simulink model "TST_CrCtl_StTrans"  (R2016b)
settings: Solver=FixedStepDiscrete  StartTime=0.0  StopTime=simTime  FixedStep=sampleTime  RelTol=1e-3
values from neighbouring files (symbols this model uses):
  testCase = 1    [initTST_CrCtl_StTrans_001.m]    (also in initTST_CrCtl_StTrans_002.m = 2; initTST_CrCtl_StTrans_003.m = 3; initTST_CrCtl_StTrans_004.m = 4; initTST_CrCtl_StTrans_005.m = 5)
libraries: simulink x46, UnitTest_Lib x5
(part 1 of 2)
settings Model: Creator=shiliwei  LastModifiedBy=shiliwei
settings DebuggingCC: SignalRangeChecking=error

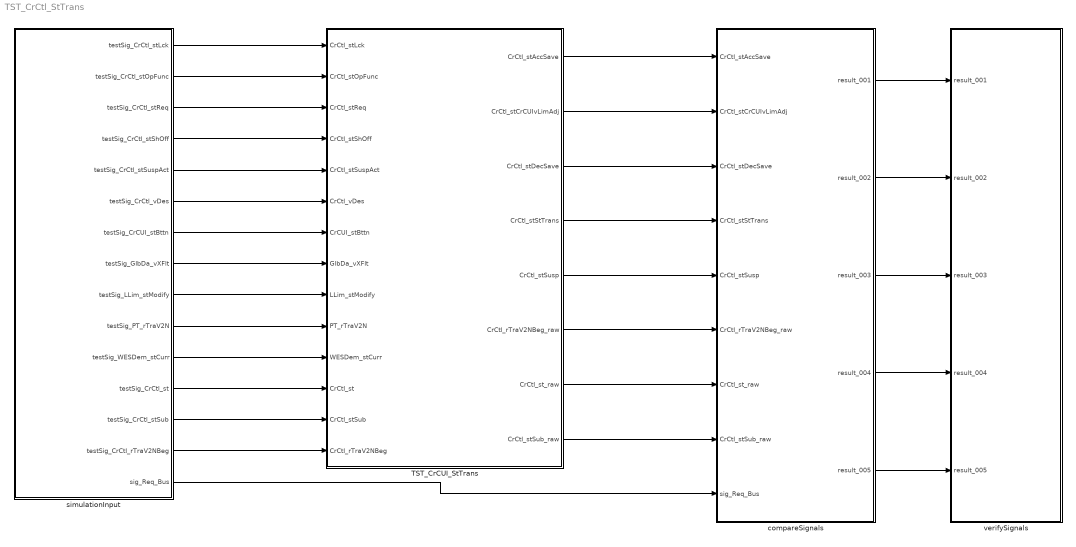
== system TST_CrCtl_StTrans ==
  TST_CrCUI_StTrans : Subsystem
  compareSignals : Subsystem
  simulationInput : Subsystem
  verifySignals : Subsystem
  wires:
  simulationInput/1(testSig_CrCtl_stLck) -> TST_CrCUI_StTrans/1(CrCtl_stLck)
  simulationInput/2(testSig_CrCtl_stOpFunc) -> TST_CrCUI_StTrans/2(CrCtl_stOpFunc)
  simulationInput/3(testSig_CrCtl_stReq) -> TST_CrCUI_StTrans/3(CrCtl_stReq)
  simulationInput/4(testSig_CrCtl_stShOff) -> TST_CrCUI_StTrans/4(CrCtl_stShOff)
  simulationInput/5(testSig_CrCtl_stSuspAct) -> TST_CrCUI_StTrans/5(CrCtl_stSuspAct)
  simulationInput/6(testSig_CrCtl_vDes) -> TST_CrCUI_StTrans/6(CrCtl_vDes)
  simulationInput/7(testSig_CrCUI_stBttn) -> TST_CrCUI_StTrans/7(CrCUI_stBttn)
  simulationInput/8(testSig_GlbDa_vXFlt) -> TST_CrCUI_StTrans/8(GlbDa_vXFlt)
  simulationInput/9(testSig_LLim_stModify) -> TST_CrCUI_StTrans/9(LLim_stModify)
  simulationInput/10(testSig_PT_rTraV2N) -> TST_CrCUI_StTrans/10(PT_rTraV2N)
  simulationInput/11(testSig_WESDem_stCurr) -> TST_CrCUI_StTrans/11(WESDem_stCurr)
  simulationInput/12(testSig_CrCtl_st) -> TST_CrCUI_StTrans/12(CrCtl_st)
  simulationInput/13(testSig_CrCtl_stSub) -> TST_CrCUI_StTrans/13(CrCtl_stSub)
  simulationInput/14(testSig_CrCtl_rTraV2NBeg) -> TST_CrCUI_StTrans/14(CrCtl_rTraV2NBeg)
  TST_CrCUI_StTrans/1(CrCtl_stAccSave) -> compareSignals/1(CrCtl_stAccSave)
  TST_CrCUI_StTrans/2(CrCtl_stCrCUIvLimAdj) -> compareSignals/2(CrCtl_stCrCUIvLimAdj)
  TST_CrCUI_StTrans/3(CrCtl_stDecSave) -> compareSignals/3(CrCtl_stDecSave)
  TST_CrCUI_StTrans/4(CrCtl_stStTrans) -> compareSignals/4(CrCtl_stStTrans)
  TST_CrCUI_StTrans/5(CrCtl_stSusp) -> compareSignals/5(CrCtl_stSusp)
  TST_CrCUI_StTrans/6(CrCtl_rTraV2NBeg_raw) -> compareSignals/6(CrCtl_rTraV2NBeg_raw)
  TST_CrCUI_StTrans/7(CrCtl_st_raw) -> compareSignals/7(CrCtl_st_raw)
  TST_CrCUI_StTrans/8(CrCtl_stSub_raw) -> compareSignals/8(CrCtl_stSub_raw)
  simulationInput/15(sig_Req_Bus) -> compareSignals/9(sig_Req_Bus)
  compareSignals/1(result_001) -> verifySignals/1(result_001)
  compareSignals/2(result_002) -> verifySignals/2(result_002)
  compareSignals/3(result_003) -> verifySignals/3(result_003)
  compareSignals/4(result_004) -> verifySignals/4(result_004)
  compareSignals/5(result_005) -> verifySignals/5(result_005)

== system TST_CrCtl_StTrans/TST_CrCUI_StTrans ==
  CrCtl_stLck : Inport
  CrCtl_stOpFunc : Inport  Port=2
  CrCtl_stReq : Inport  Port=3
  CrCtl_stShOff : Inport  Port=4
  CrCtl_stSuspAct : Inport  Port=5
  CrCtl_vDes : Inport  Port=6
  CrCUI_stBttn : Inport  Port=7
  GlbDa_vXFlt : Inport  Port=8
  LLim_stModify : Inport  Port=9
  PT_rTraV2N : Inport  Port=10
  WESDem_stCurr : Inport  Port=11
  CrCtl_st : Inport  Port=12
  CrCtl_stSub : Inport  Port=13
  CrCtl_rTraV2NBeg : Inport  Port=14
  CrCUI_StTrans : ModelReference  ModelNameDialog=CrCUI_StTrans  SimulationMode=Normal  ModelReferenceVersion=1.52  TriggerPortName=function  TriggerPortTriggerType=function-call  TriggerPortStatesWhenEnabling=held
  Function_Call : simulink/Ports & Subsystems/Function-Call Generator  sample_time=sampleTime  numberOfIterations=1
  CrCtl_stAccSave : Outport
  CrCtl_stCrCUIvLimAdj : Outport  Port=2
  CrCtl_stDecSave : Outport  Port=3
  CrCtl_stStTrans : Outport  Port=4
  CrCtl_stSusp : Outport  Port=5
  CrCtl_rTraV2NBeg_raw : Outport  Port=6
  CrCtl_st_raw : Outport  Port=7
  CrCtl_stSub_raw : Outport  Port=8
  wires:
  Function_Call/1 -> CrCUI_StTrans/Trigger
  CrCtl_stLck/1 -> CrCUI_StTrans/1
  CrCtl_stOpFunc/1 -> CrCUI_StTrans/2
  CrCtl_stReq/1 -> CrCUI_StTrans/3
  CrCtl_stShOff/1 -> CrCUI_StTrans/4
  CrCtl_stSuspAct/1 -> CrCUI_StTrans/5
  CrCtl_vDes/1 -> CrCUI_StTrans/6
  CrCUI_stBttn/1 -> CrCUI_StTrans/7
  GlbDa_vXFlt/1 -> CrCUI_StTrans/8
  LLim_stModify/1 -> CrCUI_StTrans/9
  PT_rTraV2N/1 -> CrCUI_StTrans/10
  WESDem_stCurr/1 -> CrCUI_StTrans/11
  CrCtl_st/1 -> CrCUI_StTrans/12
  CrCtl_stSub/1 -> CrCUI_StTrans/13
  CrCtl_rTraV2NBeg/1 -> CrCUI_StTrans/14
  CrCUI_StTrans/1 -> CrCtl_stAccSave/1
  CrCUI_StTrans/2 -> CrCtl_stCrCUIvLimAdj/1
  CrCUI_StTrans/3 -> CrCtl_stDecSave/1
  CrCUI_StTrans/4 -> CrCtl_stStTrans/1
  CrCUI_StTrans/5 -> CrCtl_stSusp/1
  CrCUI_StTrans/6 -> CrCtl_rTraV2NBeg_raw/1
  CrCUI_StTrans/7 -> CrCtl_st_raw/1
  CrCUI_StTrans/8 -> CrCtl_stSub_raw/1

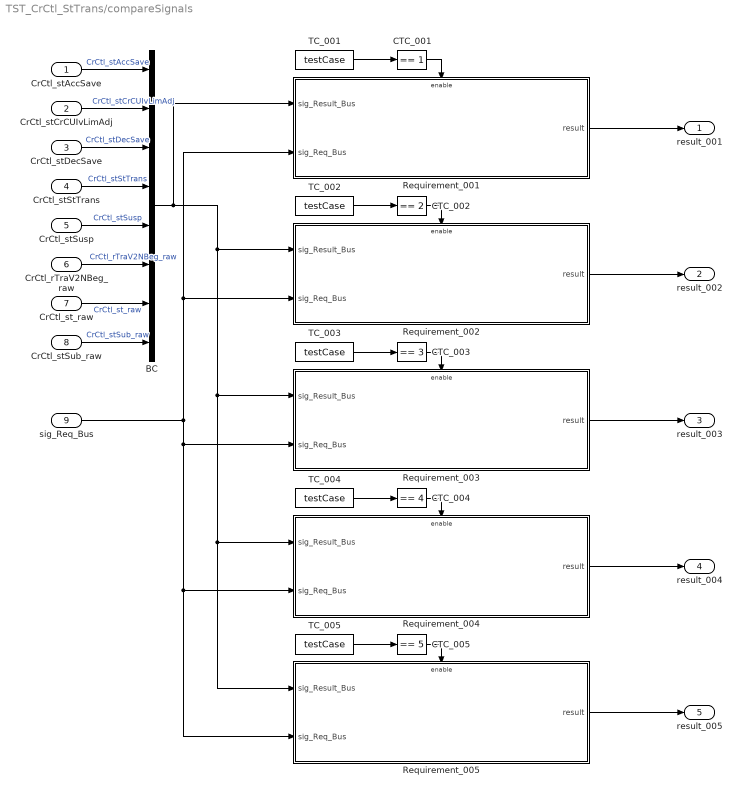
== system TST_CrCtl_StTrans/compareSignals ==
  CrCtl_stAccSave : Inport
  CrCtl_stCrCUIvLimAdj : Inport  Port=2
  CrCtl_stDecSave : Inport  Port=3
  CrCtl_stStTrans : Inport  Port=4
  CrCtl_stSusp : Inport  Port=5
  CrCtl_rTraV2NBeg_raw : Inport  Port=6
  CrCtl_st_raw : Inport  Port=7
  CrCtl_stSub_raw : Inport  Port=8
  sig_Req_Bus : Inport  Port=9
  BC : BusCreator  Inputs=8
  CTC_001 : simulink/Logic and Bit Operations/Compare To Constant  relop===  const=1  OutDataTypeStr=boolean
  CTC_002 : simulink/Logic and Bit Operations/Compare To Constant  relop===  const=2  OutDataTypeStr=boolean
  CTC_003 : simulink/Logic and Bit Operations/Compare To Constant  relop===  const=3  OutDataTypeStr=boolean
  CTC_004 : simulink/Logic and Bit Operations/Compare To Constant  relop===  const=4  OutDataTypeStr=boolean
  CTC_005 : simulink/Logic and Bit Operations/Compare To Constant  relop===  const=5  OutDataTypeStr=boolean
  Requirement_001 : Subsystem
  Requirement_002 : Subsystem
  Requirement_003 : Subsystem
  Requirement_004 : Subsystem
  Requirement_005 : Subsystem
  TC_001 : Constant  Value=testCase
  TC_002 : Constant  Value=testCase
  TC_003 : Constant  Value=testCase
  TC_004 : Constant  Value=testCase
  TC_005 : Constant  Value=testCase
  result_001 : Outport
  result_002 : Outport  Port=2
  result_003 : Outport  Port=3
  result_004 : Outport  Port=4
  result_005 : Outport  Port=5
  wires:
  CrCtl_stAccSave/1 -> BC/1  "CrCtl_stAccSave"
  CrCtl_stCrCUIvLimAdj/1 -> BC/2  "CrCtl_stCrCUIvLimAdj"
  CrCtl_stDecSave/1 -> BC/3  "CrCtl_stDecSave"
  CrCtl_stStTrans/1 -> BC/4  "CrCtl_stStTrans"
  CrCtl_stSusp/1 -> BC/5  "CrCtl_stSusp"
  CrCtl_rTraV2NBeg_raw/1 -> BC/6  "CrCtl_rTraV2NBeg_raw"
  CrCtl_st_raw/1 -> BC/7  "CrCtl_st_raw"
  CrCtl_stSub_raw/1 -> BC/8  "CrCtl_stSub_raw"
  TC_001/1 -> CTC_001/1
  CTC_001/1 -> Requirement_001/Enable
  sig_Req_Bus/1 -> Requirement_004/2(sig_Req_Bus), Requirement_005/2(sig_Req_Bus), Requirement_003/2(sig_Req_Bus), Requirement_001/2(sig_Req_Bus), Requirement_002/2(sig_Req_Bus)
  BC/1 -> Requirement_004/1(sig_Result_Bus), Requirement_005/1(sig_Result_Bus), Requirement_003/1(sig_Result_Bus), Requirement_002/1(sig_Result_Bus), Requirement_001/1(sig_Result_Bus)
  Requirement_001/1(result) -> result_001/1
  TC_002/1 -> CTC_002/1
  CTC_002/1 -> Requirement_002/Enable
  Requirement_002/1(result) -> result_002/1
  TC_003/1 -> CTC_003/1
  CTC_003/1 -> Requirement_003/Enable
  Requirement_003/1(result) -> result_003/1
  TC_004/1 -> CTC_004/1
  CTC_004/1 -> Requirement_004/Enable
  Requirement_004/1(result) -> result_004/1
  TC_005/1 -> CTC_005/1
  CTC_005/1 -> Requirement_005/Enable
  Requirement_005/1(result) -> result_005/1

== system TST_CrCtl_StTrans/simulationInput ==
  BS : BusSelector  OutputSignals=testSig_CrCtl_stLck,testSig_CrCtl_stOpFunc,testSig_CrCtl_stReq,testSig_CrCtl_stShOff,testSig_CrCtl_stSuspAct,testSig_CrCtl_vDes,testSig_CrCUI_stBttn,testSig_GlbDa_vXFlt,testSig_LLim_stModify,testSig_PT_rTraV2N,testSig_WESDem_stCurr,testSig_CrCtl_st,testSig_CrCtl_stSub,testSig_CrCtl_rTraV2NBeg
  MPSw : MultiPortSwitch  Inputs=5  SaturateOnIntegerOverflow=on  InputSameDT=on
  TestCase : Constant  Value=testCase
  testSignals_R001 : Subsystem
  testSignals_R002 : Subsystem
  testSignals_R003 : Subsystem
  testSignals_R004 : Subsystem
  testSignals_R005 : Subsystem
  testSig_CrCtl_stLck : Outport
  testSig_CrCtl_stOpFunc : Outport  Port=2
  testSig_CrCtl_stReq : Outport  Port=3
  testSig_CrCtl_stShOff : Outport  Port=4
  testSig_CrCtl_stSuspAct : Outport  Port=5
  testSig_CrCtl_vDes : Outport  Port=6
  testSig_CrCUI_stBttn : Outport  Port=7
  testSig_GlbDa_vXFlt : Outport  Port=8
  testSig_LLim_stModify : Outport  Port=9
  testSig_PT_rTraV2N : Outport  Port=10
  testSig_WESDem_stCurr : Outport  Port=11
  testSig_CrCtl_st : Outport  Port=12
  testSig_CrCtl_stSub : Outport  Port=13
  testSig_CrCtl_rTraV2NBeg : Outport  Port=14
  sig_Req_Bus : Outport  Port=15
  wires:
  BS/1 -> testSig_CrCtl_stLck/1  "<testSig_CrCtl_stLck>"
  BS/2 -> testSig_CrCtl_stOpFunc/1  "<testSig_CrCtl_stOpFunc>"
  BS/3 -> testSig_CrCtl_stReq/1  "<testSig_CrCtl_stReq>"
  BS/4 -> testSig_CrCtl_stShOff/1  "<testSig_CrCtl_stShOff>"
  BS/5 -> testSig_CrCtl_stSuspAct/1  "<testSig_CrCtl_stSuspAct>"
  BS/6 -> testSig_CrCtl_vDes/1  "<testSig_CrCtl_vDes>"
  BS/7 -> testSig_CrCUI_stBttn/1  "<testSig_CrCUI_stBttn>"
  BS/8 -> testSig_GlbDa_vXFlt/1  "<testSig_GlbDa_vXFlt>"
  BS/9 -> testSig_LLim_stModify/1  "<testSig_LLim_stModify>"
  BS/10 -> testSig_PT_rTraV2N/1  "<testSig_PT_rTraV2N>"
  BS/11 -> testSig_WESDem_stCurr/1  "<testSig_WESDem_stCurr>"
  BS/12 -> testSig_CrCtl_st/1  "<testSig_CrCtl_st>"
  BS/13 -> testSig_CrCtl_stSub/1  "<testSig_CrCtl_stSub>"
  BS/14 -> testSig_CrCtl_rTraV2NBeg/1  "<testSig_CrCtl_rTraV2NBeg>"
  MPSw/1 -> BS/1, sig_Req_Bus/1
  TestCase/1 -> MPSw/1
  testSignals_R001/1(testSignals) -> MPSw/2
  testSignals_R002/1(testSignals) -> MPSw/3
  testSignals_R003/1(testSignals) -> MPSw/4
  testSignals_R004/1(testSignals) -> MPSw/5
  testSignals_R005/1(testSignals) -> MPSw/6

== system TST_CrCtl_StTrans/verifySignals ==
  result_001 : Inport
  result_002 : Inport  Port=2
  result_003 : Inport  Port=3
  result_004 : Inport  Port=4
  result_005 : Inport  Port=5
  Assertion_001 : Assertion  Enabled=off
  Assertion_002 : Assertion  Enabled=off
  Assertion_003 : Assertion  Enabled=off
  Assertion_004 : Assertion  Enabled=off
  Assertion_005 : Assertion  Enabled=off
  wires:
  result_001/1 -> Assertion_001/1
  result_002/1 -> Assertion_002/1
  result_003/1 -> Assertion_003/1
  result_004/1 -> Assertion_004/1
  result_005/1 -> Assertion_005/1

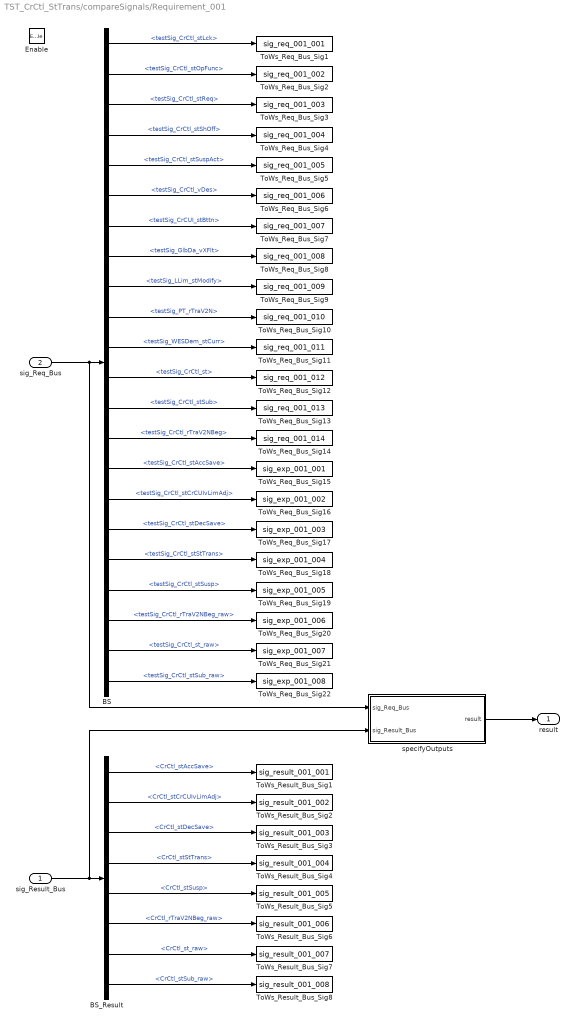
== system TST_CrCtl_StTrans/compareSignals/Requirement_001 ==
  sig_Result_Bus : Inport
  sig_Req_Bus : Inport  Port=2
  Enable : EnablePort
  BS : BusSelector  OutputSignals=testSig_CrCtl_stLck,testSig_CrCtl_stOpFunc,testSig_CrCtl_stReq,testSig_CrCtl_stShOff,testSig_CrCtl_stSuspAct,testSig_CrCtl_vDes,testSig_CrCUI_stBttn,testSig_GlbDa_vXFlt,testSig_LLim_stModify,testSig_PT_rTraV2N,testSig_WESDem_stCurr,testSig_CrCtl_st,testSig_CrCtl_stSub,testSig_CrCtl_rTraV2NBeg,testSig_CrCtl_stAccSave,testSig_CrCtl_stCrCUIvLimAdj,testSig_CrCtl_stDecSave,testSig_CrCtl_stStTrans,testSig_CrCtl_stSusp,testSig_CrCtl_rTraV2NBeg_raw,testSig_CrCtl_st_raw,testSig_CrCtl_stSub_raw
  BS_Result : BusSelector  OutputSignals=CrCtl_stAccSave,CrCtl_stCrCUIvLimAdj,CrCtl_stDecSave,CrCtl_stStTrans,CrCtl_stSusp,CrCtl_rTraV2NBeg_raw,CrCtl_st_raw,CrCtl_stSub_raw
  ToWs_Req_Bus_Sig1 : ToWorkspace  VariableName=sig_req_001_001  SaveFormat=Structure With Time
  ToWs_Req_Bus_Sig10 : ToWorkspace  VariableName=sig_req_001_010  SaveFormat=Structure With Time
  ToWs_Req_Bus_Sig11 : ToWorkspace  VariableName=sig_req_001_011  SaveFormat=Structure With Time
  ToWs_Req_Bus_Sig12 : ToWorkspace  VariableName=sig_req_001_012  SaveFormat=Structure With Time
  ToWs_Req_Bus_Sig13 : ToWorkspace  VariableName=sig_req_001_013  SaveFormat=Structure With Time
  ToWs_Req_Bus_Sig14 : ToWorkspace  VariableName=sig_req_001_014  SaveFormat=Structure With Time
  ToWs_Req_Bus_Sig15 : ToWorkspace  VariableName=sig_exp_001_001  SaveFormat=Structure With Time
  ToWs_Req_Bus_Sig16 : ToWorkspace  VariableName=sig_exp_001_002  SaveFormat=Structure With Time
  ToWs_Req_Bus_Sig17 : ToWorkspace  VariableName=sig_exp_001_003  SaveFormat=Structure With Time
  ToWs_Req_Bus_Sig18 : ToWorkspace  VariableName=sig_exp_001_004  SaveFormat=Structure With Time
  ToWs_Req_Bus_Sig19 : ToWorkspace  VariableName=sig_exp_001_005  SaveFormat=Structure With Time
  ToWs_Req_Bus_Sig2 : ToWorkspace  VariableName=sig_req_001_002  SaveFormat=Structure With Time
  ToWs_Req_Bus_Sig20 : ToWorkspace  VariableName=sig_exp_001_006  SaveFormat=Structure With Time
  ToWs_Req_Bus_Sig21 : ToWorkspace  VariableName=sig_exp_001_007  SaveFormat=Structure With Time
  ToWs_Req_Bus_Sig22 : ToWorkspace  VariableName=sig_exp_001_008  SaveFormat=Structure With Time
  ToWs_Req_Bus_Sig3 : ToWorkspace  VariableName=sig_req_001_003  SaveFormat=Structure With Time
  ToWs_Req_Bus_Sig4 : ToWorkspace  VariableName=sig_req_001_004  SaveFormat=Structure With Time
  ToWs_Req_Bus_Sig5 : ToWorkspace  VariableName=sig_req_001_005  SaveFormat=Structure With Time
  ToWs_Req_Bus_Sig6 : ToWorkspace  VariableName=sig_req_001_006  SaveFormat=Structure With Time
  ToWs_Req_Bus_Sig7 : ToWorkspace  VariableName=sig_req_001_007  SaveFormat=Structure With Time
  ToWs_Req_Bus_Sig8 : ToWorkspace  VariableName=sig_req_001_008  SaveFormat=Structure With Time
  ToWs_Req_Bus_Sig9 : ToWorkspace  VariableName=sig_req_001_009  SaveFormat=Structure With Time
  ToWs_Result_Bus_Sig1 : ToWorkspace  VariableName=sig_result_001_001  SaveFormat=Structure With Time
  ToWs_Result_Bus_Sig2 : ToWorkspace  VariableName=sig_result_001_002  SaveFormat=Structure With Time
  ToWs_Result_Bus_Sig3 : ToWorkspace  VariableName=sig_result_001_003  SaveFormat=Structure With Time
  ToWs_Result_Bus_Sig4 : ToWorkspace  VariableName=sig_result_001_004  SaveFormat=Structure With Time
  ToWs_Result_Bus_Sig5 : ToWorkspace  VariableName=sig_result_001_005  SaveFormat=Structure With Time
  ToWs_Result_Bus_Sig6 : ToWorkspace  VariableName=sig_result_001_006  SaveFormat=Structure With Time
  ToWs_Result_Bus_Sig7 : ToWorkspace  VariableName=sig_result_001_007  SaveFormat=Structure With Time
  ToWs_Result_Bus_Sig8 : ToWorkspace  VariableName=sig_result_001_008  SaveFormat=Structure With Time
  specifyOutputs : Subsystem
  result : Outport
  wires:
  sig_Req_Bus/1 -> BS/1, specifyOutputs/1(sig_Req_Bus)
  BS/1 -> ToWs_Req_Bus_Sig1/1  "<testSig_CrCtl_stLck>"
  BS/2 -> ToWs_Req_Bus_Sig2/1  "<testSig_CrCtl_stOpFunc>"
  BS/3 -> ToWs_Req_Bus_Sig3/1  "<testSig_CrCtl_stReq>"
  BS/4 -> ToWs_Req_Bus_Sig4/1  "<testSig_CrCtl_stShOff>"
  BS/5 -> ToWs_Req_Bus_Sig5/1  "<testSig_CrCtl_stSuspAct>"
  BS/6 -> ToWs_Req_Bus_Sig6/1  "<testSig_CrCtl_vDes>"
  BS/7 -> ToWs_Req_Bus_Sig7/1  "<testSig_CrCUI_stBttn>"
  BS/8 -> ToWs_Req_Bus_Sig8/1  "<testSig_GlbDa_vXFlt>"
  BS/9 -> ToWs_Req_Bus_Sig9/1  "<testSig_LLim_stModify>"
  BS/10 -> ToWs_Req_Bus_Sig10/1  "<testSig_PT_rTraV2N>"
  BS/11 -> ToWs_Req_Bus_Sig11/1  "<testSig_WESDem_stCurr>"
  BS/12 -> ToWs_Req_Bus_Sig12/1  "<testSig_CrCtl_st>"
  BS/13 -> ToWs_Req_Bus_Sig13/1  "<testSig_CrCtl_stSub>"
  BS/14 -> ToWs_Req_Bus_Sig14/1  "<testSig_CrCtl_rTraV2NBeg>"
  BS/15 -> ToWs_Req_Bus_Sig15/1  "<testSig_CrCtl_stAccSave>"
  BS/16 -> ToWs_Req_Bus_Sig16/1  "<testSig_CrCtl_stCrCUIvLimAdj>"
  BS/17 -> ToWs_Req_Bus_Sig17/1  "<testSig_CrCtl_stDecSave>"
  BS/18 -> ToWs_Req_Bus_Sig18/1  "<testSig_CrCtl_stStTrans>"
  BS/19 -> ToWs_Req_Bus_Sig19/1  "<testSig_CrCtl_stSusp>"
  BS/20 -> ToWs_Req_Bus_Sig20/1  "<testSig_CrCtl_rTraV2NBeg_raw>"
  BS/21 -> ToWs_Req_Bus_Sig21/1  "<testSig_CrCtl_st_raw>"
  BS/22 -> ToWs_Req_Bus_Sig22/1  "<testSig_CrCtl_stSub_raw>"
  sig_Result_Bus/1 -> BS_Result/1, specifyOutputs/2(sig_Result_Bus)
  BS_Result/1 -> ToWs_Result_Bus_Sig1/1  "<CrCtl_stAccSave>"
  BS_Result/2 -> ToWs_Result_Bus_Sig2/1  "<CrCtl_stCrCUIvLimAdj>"
  BS_Result/3 -> ToWs_Result_Bus_Sig3/1  "<CrCtl_stDecSave>"
  BS_Result/4 -> ToWs_Result_Bus_Sig4/1  "<CrCtl_stStTrans>"
  BS_Result/5 -> ToWs_Result_Bus_Sig5/1  "<CrCtl_stSusp>"
  BS_Result/6 -> ToWs_Result_Bus_Sig6/1  "<CrCtl_rTraV2NBeg_raw>"
  BS_Result/7 -> ToWs_Result_Bus_Sig7/1  "<CrCtl_st_raw>"
  BS_Result/8 -> ToWs_Result_Bus_Sig8/1  "<CrCtl_stSub_raw>"
  specifyOutputs/1(result) -> result/1

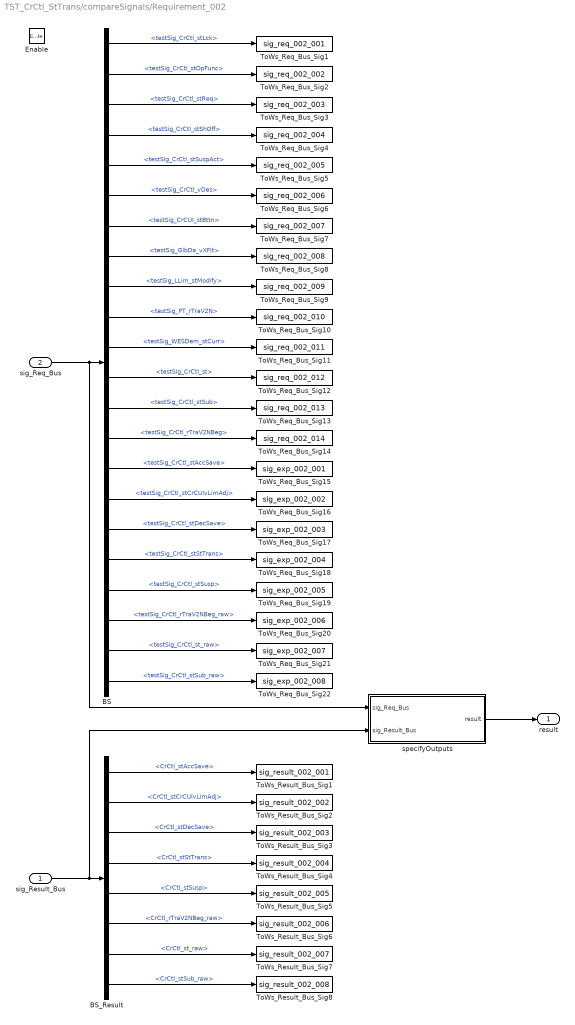
== system TST_CrCtl_StTrans/compareSignals/Requirement_002 ==
  sig_Result_Bus : Inport
  sig_Req_Bus : Inport  Port=2
  Enable : EnablePort
  BS : BusSelector  OutputSignals=testSig_CrCtl_stLck,testSig_CrCtl_stOpFunc,testSig_CrCtl_stReq,testSig_CrCtl_stShOff,testSig_CrCtl_stSuspAct,testSig_CrCtl_vDes,testSig_CrCUI_stBttn,testSig_GlbDa_vXFlt,testSig_LLim_stModify,testSig_PT_rTraV2N,testSig_WESDem_stCurr,testSig_CrCtl_st,testSig_CrCtl_stSub,testSig_CrCtl_rTraV2NBeg,testSig_CrCtl_stAccSave,testSig_CrCtl_stCrCUIvLimAdj,testSig_CrCtl_stDecSave,testSig_CrCtl_stStTrans,testSig_CrCtl_stSusp,testSig_CrCtl_rTraV2NBeg_raw,testSig_CrCtl_st_raw,testSig_CrCtl_stSub_raw
  BS_Result : BusSelector  OutputSignals=CrCtl_stAccSave,CrCtl_stCrCUIvLimAdj,CrCtl_stDecSave,CrCtl_stStTrans,CrCtl_stSusp,CrCtl_rTraV2NBeg_raw,CrCtl_st_raw,CrCtl_stSub_raw
  ToWs_Req_Bus_Sig1 : ToWorkspace  VariableName=sig_req_002_001  SaveFormat=Structure With Time
  ToWs_Req_Bus_Sig10 : ToWorkspace  VariableName=sig_req_002_010  SaveFormat=Structure With Time
  ToWs_Req_Bus_Sig11 : ToWorkspace  VariableName=sig_req_002_011  SaveFormat=Structure With Time
  ToWs_Req_Bus_Sig12 : ToWorkspace  VariableName=sig_req_002_012  SaveFormat=Structure With Time
  ToWs_Req_Bus_Sig13 : ToWorkspace  VariableName=sig_req_002_013  SaveFormat=Structure With Time
  ToWs_Req_Bus_Sig14 : ToWorkspace  VariableName=sig_req_002_014  SaveFormat=Structure With Time
  ToWs_Req_Bus_Sig15 : ToWorkspace  VariableName=sig_exp_002_001  SaveFormat=Structure With Time
  ToWs_Req_Bus_Sig16 : ToWorkspace  VariableName=sig_exp_002_002  SaveFormat=Structure With Time
  ToWs_Req_Bus_Sig17 : ToWorkspace  VariableName=sig_exp_002_003  SaveFormat=Structure With Time
  ToWs_Req_Bus_Sig18 : ToWorkspace  VariableName=sig_exp_002_004  SaveFormat=Structure With Time
  ToWs_Req_Bus_Sig19 : ToWorkspace  VariableName=sig_exp_002_005  SaveFormat=Structure With Time
  ToWs_Req_Bus_Sig2 : ToWorkspace  VariableName=sig_req_002_002  SaveFormat=Structure With Time
  ToWs_Req_Bus_Sig20 : ToWorkspace  VariableName=sig_exp_002_006  SaveFormat=Structure With Time
  ToWs_Req_Bus_Sig21 : ToWorkspace  VariableName=sig_exp_002_007  SaveFormat=Structure With Time
  ToWs_Req_Bus_Sig22 : ToWorkspace  VariableName=sig_exp_002_008  SaveFormat=Structure With Time
  ToWs_Req_Bus_Sig3 : ToWorkspace  VariableName=sig_req_002_003  SaveFormat=Structure With Time
  ToWs_Req_Bus_Sig4 : ToWorkspace  VariableName=sig_req_002_004  SaveFormat=Structure With Time
  ToWs_Req_Bus_Sig5 : ToWorkspace  VariableName=sig_req_002_005  SaveFormat=Structure With Time
  ToWs_Req_Bus_Sig6 : ToWorkspace  VariableName=sig_req_002_006  SaveFormat=Structure With Time
  ToWs_Req_Bus_Sig7 : ToWorkspace  VariableName=sig_req_002_007  SaveFormat=Structure With Time
  ToWs_Req_Bus_Sig8 : ToWorkspace  VariableName=sig_req_002_008  SaveFormat=Structure With Time
  ToWs_Req_Bus_Sig9 : ToWorkspace  VariableName=sig_req_002_009  SaveFormat=Structure With Time
  ToWs_Result_Bus_Sig1 : ToWorkspace  VariableName=sig_result_002_001  SaveFormat=Structure With Time
  ToWs_Result_Bus_Sig2 : ToWorkspace  VariableName=sig_result_002_002  SaveFormat=Structure With Time
  ToWs_Result_Bus_Sig3 : ToWorkspace  VariableName=sig_result_002_003  SaveFormat=Structure With Time
  ToWs_Result_Bus_Sig4 : ToWorkspace  VariableName=sig_result_002_004  SaveFormat=Structure With Time
  ToWs_Result_Bus_Sig5 : ToWorkspace  VariableName=sig_result_002_005  SaveFormat=Structure With Time
  ToWs_Result_Bus_Sig6 : ToWorkspace  VariableName=sig_result_002_006  SaveFormat=Structure With Time
  ToWs_Result_Bus_Sig7 : ToWorkspace  VariableName=sig_result_002_007  SaveFormat=Structure With Time
  ToWs_Result_Bus_Sig8 : ToWorkspace  VariableName=sig_result_002_008  SaveFormat=Structure With Time
  specifyOutputs : Subsystem
  result : Outport
  wires:
  sig_Req_Bus/1 -> BS/1, specifyOutputs/1(sig_Req_Bus)
  BS/1 -> ToWs_Req_Bus_Sig1/1  "<testSig_CrCtl_stLck>"
  BS/2 -> ToWs_Req_Bus_Sig2/1  "<testSig_CrCtl_stOpFunc>"
  BS/3 -> ToWs_Req_Bus_Sig3/1  "<testSig_CrCtl_stReq>"
  BS/4 -> ToWs_Req_Bus_Sig4/1  "<testSig_CrCtl_stShOff>"
  BS/5 -> ToWs_Req_Bus_Sig5/1  "<testSig_CrCtl_stSuspAct>"
  BS/6 -> ToWs_Req_Bus_Sig6/1  "<testSig_CrCtl_vDes>"
  BS/7 -> ToWs_Req_Bus_Sig7/1  "<testSig_CrCUI_stBttn>"
  BS/8 -> ToWs_Req_Bus_Sig8/1  "<testSig_GlbDa_vXFlt>"
  BS/9 -> ToWs_Req_Bus_Sig9/1  "<testSig_LLim_stModify>"
  BS/10 -> ToWs_Req_Bus_Sig10/1  "<testSig_PT_rTraV2N>"
  BS/11 -> ToWs_Req_Bus_Sig11/1  "<testSig_WESDem_stCurr>"
  BS/12 -> ToWs_Req_Bus_Sig12/1  "<testSig_CrCtl_st>"
  BS/13 -> ToWs_Req_Bus_Sig13/1  "<testSig_CrCtl_stSub>"
  BS/14 -> ToWs_Req_Bus_Sig14/1  "<testSig_CrCtl_rTraV2NBeg>"
  BS/15 -> ToWs_Req_Bus_Sig15/1  "<testSig_CrCtl_stAccSave>"
  BS/16 -> ToWs_Req_Bus_Sig16/1  "<testSig_CrCtl_stCrCUIvLimAdj>"
  BS/17 -> ToWs_Req_Bus_Sig17/1  "<testSig_CrCtl_stDecSave>"
  BS/18 -> ToWs_Req_Bus_Sig18/1  "<testSig_CrCtl_stStTrans>"
  BS/19 -> ToWs_Req_Bus_Sig19/1  "<testSig_CrCtl_stSusp>"
  BS/20 -> ToWs_Req_Bus_Sig20/1  "<testSig_CrCtl_rTraV2NBeg_raw>"
  BS/21 -> ToWs_Req_Bus_Sig21/1  "<testSig_CrCtl_st_raw>"
  BS/22 -> ToWs_Req_Bus_Sig22/1  "<testSig_CrCtl_stSub_raw>"
  sig_Result_Bus/1 -> BS_Result/1, specifyOutputs/2(sig_Result_Bus)
  BS_Result/1 -> ToWs_Result_Bus_Sig1/1  "<CrCtl_stAccSave>"
  BS_Result/2 -> ToWs_Result_Bus_Sig2/1  "<CrCtl_stCrCUIvLimAdj>"
  BS_Result/3 -> ToWs_Result_Bus_Sig3/1  "<CrCtl_stDecSave>"
  BS_Result/4 -> ToWs_Result_Bus_Sig4/1  "<CrCtl_stStTrans>"
  BS_Result/5 -> ToWs_Result_Bus_Sig5/1  "<CrCtl_stSusp>"
  BS_Result/6 -> ToWs_Result_Bus_Sig6/1  "<CrCtl_rTraV2NBeg_raw>"
  BS_Result/7 -> ToWs_Result_Bus_Sig7/1  "<CrCtl_st_raw>"
  BS_Result/8 -> ToWs_Result_Bus_Sig8/1  "<CrCtl_stSub_raw>"
  specifyOutputs/1(result) -> result/1

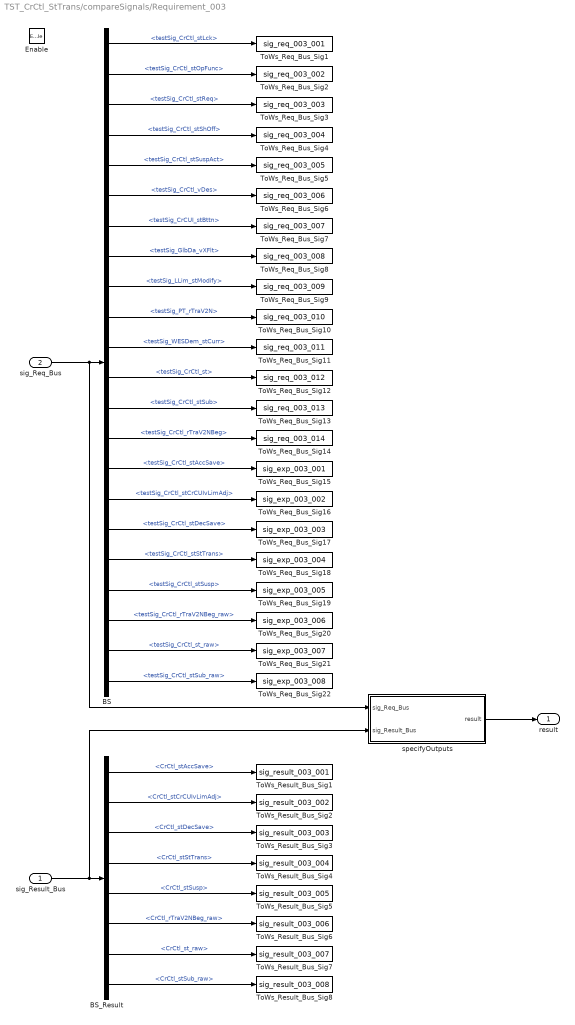
== system TST_CrCtl_StTrans/compareSignals/Requirement_003 ==
  sig_Result_Bus : Inport
  sig_Req_Bus : Inport  Port=2
  Enable : EnablePort
  BS : BusSelector  OutputSignals=testSig_CrCtl_stLck,testSig_CrCtl_stOpFunc,testSig_CrCtl_stReq,testSig_CrCtl_stShOff,testSig_CrCtl_stSuspAct,testSig_CrCtl_vDes,testSig_CrCUI_stBttn,testSig_GlbDa_vXFlt,testSig_LLim_stModify,testSig_PT_rTraV2N,testSig_WESDem_stCurr,testSig_CrCtl_st,testSig_CrCtl_stSub,testSig_CrCtl_rTraV2NBeg,testSig_CrCtl_stAccSave,testSig_CrCtl_stCrCUIvLimAdj,testSig_CrCtl_stDecSave,testSig_CrCtl_stStTrans,testSig_CrCtl_stSusp,testSig_CrCtl_rTraV2NBeg_raw,testSig_CrCtl_st_raw,testSig_CrCtl_stSub_raw
  BS_Result : BusSelector  OutputSignals=CrCtl_stAccSave,CrCtl_stCrCUIvLimAdj,CrCtl_stDecSave,CrCtl_stStTrans,CrCtl_stSusp,CrCtl_rTraV2NBeg_raw,CrCtl_st_raw,CrCtl_stSub_raw
  ToWs_Req_Bus_Sig1 : ToWorkspace  VariableName=sig_req_003_001  SaveFormat=Structure With Time
  ToWs_Req_Bus_Sig10 : ToWorkspace  VariableName=sig_req_003_010  SaveFormat=Structure With Time
  ToWs_Req_Bus_Sig11 : ToWorkspace  VariableName=sig_req_003_011  SaveFormat=Structure With Time
  ToWs_Req_Bus_Sig12 : ToWorkspace  VariableName=sig_req_003_012  SaveFormat=Structure With Time
  ToWs_Req_Bus_Sig13 : ToWorkspace  VariableName=sig_req_003_013  SaveFormat=Structure With Time
  ToWs_Req_Bus_Sig14 : ToWorkspace  VariableName=sig_req_003_014  SaveFormat=Structure With Time
  ToWs_Req_Bus_Sig15 : ToWorkspace  VariableName=sig_exp_003_001  SaveFormat=Structure With Time
  ToWs_Req_Bus_Sig16 : ToWorkspace  VariableName=sig_exp_003_002  SaveFormat=Structure With Time
  ToWs_Req_Bus_Sig17 : ToWorkspace  VariableName=sig_exp_003_003  SaveFormat=Structure With Time
  ToWs_Req_Bus_Sig18 : ToWorkspace  VariableName=sig_exp_003_004  SaveFormat=Structure With Time
  ToWs_Req_Bus_Sig19 : ToWorkspace  VariableName=sig_exp_003_005  SaveFormat=Structure With Time
  ToWs_Req_Bus_Sig2 : ToWorkspace  VariableName=sig_req_003_002  SaveFormat=Structure With Time
  ToWs_Req_Bus_Sig20 : ToWorkspace  VariableName=sig_exp_003_006  SaveFormat=Structure With Time
  ToWs_Req_Bus_Sig21 : ToWorkspace  VariableName=sig_exp_003_007  SaveFormat=Structure With Time
  ToWs_Req_Bus_Sig22 : ToWorkspace  VariableName=sig_exp_003_008  SaveFormat=Structure With Time
  ToWs_Req_Bus_Sig3 : ToWorkspace  VariableName=sig_req_003_003  SaveFormat=Structure With Time
  ToWs_Req_Bus_Sig4 : ToWorkspace  VariableName=sig_req_003_004  SaveFormat=Structure With Time
  ToWs_Req_Bus_Sig5 : ToWorkspace  VariableName=sig_req_003_005  SaveFormat=Structure With Time
  ToWs_Req_Bus_Sig6 : ToWorkspace  VariableName=sig_req_003_006  SaveFormat=Structure With Time
  ToWs_Req_Bus_Sig7 : ToWorkspace  VariableName=sig_req_003_007  SaveFormat=Structure With Time
  ToWs_Req_Bus_Sig8 : ToWorkspace  VariableName=sig_req_003_008  SaveFormat=Structure With Time
  ToWs_Req_Bus_Sig9 : ToWorkspace  VariableName=sig_req_003_009  SaveFormat=Structure With Time
  ToWs_Result_Bus_Sig1 : ToWorkspace  VariableName=sig_result_003_001  SaveFormat=Structure With Time
  ToWs_Result_Bus_Sig2 : ToWorkspace  VariableName=sig_result_003_002  SaveFormat=Structure With Time
  ToWs_Result_Bus_Sig3 : ToWorkspace  VariableName=sig_result_003_003  SaveFormat=Structure With Time
  ToWs_Result_Bus_Sig4 : ToWorkspace  VariableName=sig_result_003_004  SaveFormat=Structure With Time
  ToWs_Result_Bus_Sig5 : ToWorkspace  VariableName=sig_result_003_005  SaveFormat=Structure With Time
  ToWs_Result_Bus_Sig6 : ToWorkspace  VariableName=sig_result_003_006  SaveFormat=Structure With Time
  ToWs_Result_Bus_Sig7 : ToWorkspace  VariableName=sig_result_003_007  SaveFormat=Structure With Time
  ToWs_Result_Bus_Sig8 : ToWorkspace  VariableName=sig_result_003_008  SaveFormat=Structure With Time
  specifyOutputs : Subsystem
  result : Outport
  wires:
  sig_Req_Bus/1 -> BS/1, specifyOutputs/1(sig_Req_Bus)
  BS/1 -> ToWs_Req_Bus_Sig1/1  "<testSig_CrCtl_stLck>"
  BS/2 -> ToWs_Req_Bus_Sig2/1  "<testSig_CrCtl_stOpFunc>"
  BS/3 -> ToWs_Req_Bus_Sig3/1  "<testSig_CrCtl_stReq>"
  BS/4 -> ToWs_Req_Bus_Sig4/1  "<testSig_CrCtl_stShOff>"
  BS/5 -> ToWs_Req_Bus_Sig5/1  "<testSig_CrCtl_stSuspAct>"
  BS/6 -> ToWs_Req_Bus_Sig6/1  "<testSig_CrCtl_vDes>"
  BS/7 -> ToWs_Req_Bus_Sig7/1  "<testSig_CrCUI_stBttn>"
  BS/8 -> ToWs_Req_Bus_Sig8/1  "<testSig_GlbDa_vXFlt>"
  BS/9 -> ToWs_Req_Bus_Sig9/1  "<testSig_LLim_stModify>"
  BS/10 -> ToWs_Req_Bus_Sig10/1  "<testSig_PT_rTraV2N>"
  BS/11 -> ToWs_Req_Bus_Sig11/1  "<testSig_WESDem_stCurr>"
  BS/12 -> ToWs_Req_Bus_Sig12/1  "<testSig_CrCtl_st>"
  BS/13 -> ToWs_Req_Bus_Sig13/1  "<testSig_CrCtl_stSub>"
  BS/14 -> ToWs_Req_Bus_Sig14/1  "<testSig_CrCtl_rTraV2NBeg>"
  BS/15 -> ToWs_Req_Bus_Sig15/1  "<testSig_CrCtl_stAccSave>"
  BS/16 -> ToWs_Req_Bus_Sig16/1  "<testSig_CrCtl_stCrCUIvLimAdj>"
  BS/17 -> ToWs_Req_Bus_Sig17/1  "<testSig_CrCtl_stDecSave>"
  BS/18 -> ToWs_Req_Bus_Sig18/1  "<testSig_CrCtl_stStTrans>"
  BS/19 -> ToWs_Req_Bus_Sig19/1  "<testSig_CrCtl_stSusp>"
  BS/20 -> ToWs_Req_Bus_Sig20/1  "<testSig_CrCtl_rTraV2NBeg_raw>"
  BS/21 -> ToWs_Req_Bus_Sig21/1  "<testSig_CrCtl_st_raw>"
  BS/22 -> ToWs_Req_Bus_Sig22/1  "<testSig_CrCtl_stSub_raw>"
  sig_Result_Bus/1 -> BS_Result/1, specifyOutputs/2(sig_Result_Bus)
  BS_Result/1 -> ToWs_Result_Bus_Sig1/1  "<CrCtl_stAccSave>"
  BS_Result/2 -> ToWs_Result_Bus_Sig2/1  "<CrCtl_stCrCUIvLimAdj>"
  BS_Result/3 -> ToWs_Result_Bus_Sig3/1  "<CrCtl_stDecSave>"
  BS_Result/4 -> ToWs_Result_Bus_Sig4/1  "<CrCtl_stStTrans>"
  BS_Result/5 -> ToWs_Result_Bus_Sig5/1  "<CrCtl_stSusp>"
  BS_Result/6 -> ToWs_Result_Bus_Sig6/1  "<CrCtl_rTraV2NBeg_raw>"
  BS_Result/7 -> ToWs_Result_Bus_Sig7/1  "<CrCtl_st_raw>"
  BS_Result/8 -> ToWs_Result_Bus_Sig8/1  "<CrCtl_stSub_raw>"
  specifyOutputs/1(result) -> result/1

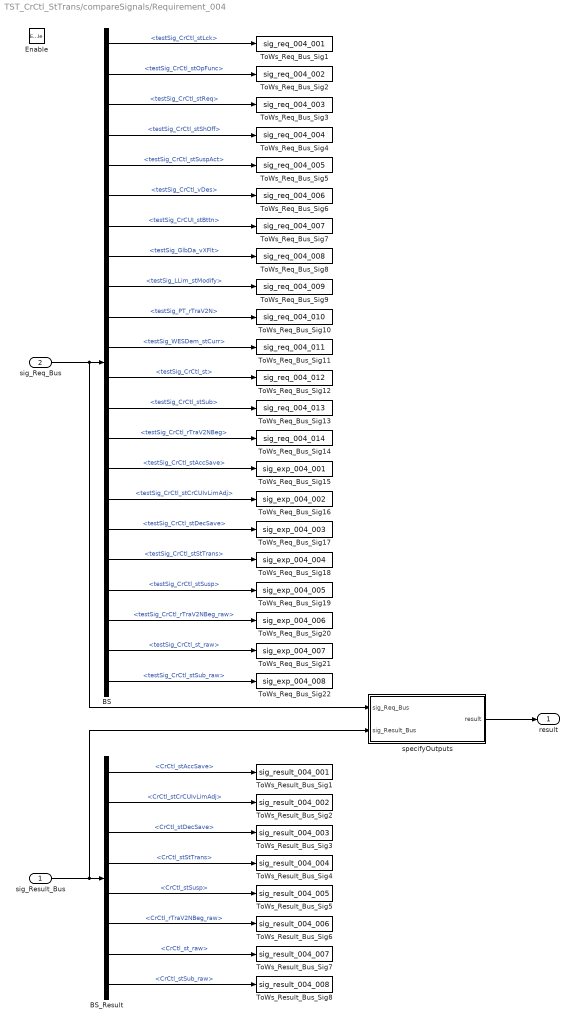
== system TST_CrCtl_StTrans/compareSignals/Requirement_004 ==
  sig_Result_Bus : Inport
  sig_Req_Bus : Inport  Port=2
  Enable : EnablePort
  BS : BusSelector  OutputSignals=testSig_CrCtl_stLck,testSig_CrCtl_stOpFunc,testSig_CrCtl_stReq,testSig_CrCtl_stShOff,testSig_CrCtl_stSuspAct,testSig_CrCtl_vDes,testSig_CrCUI_stBttn,testSig_GlbDa_vXFlt,testSig_LLim_stModify,testSig_PT_rTraV2N,testSig_WESDem_stCurr,testSig_CrCtl_st,testSig_CrCtl_stSub,testSig_CrCtl_rTraV2NBeg,testSig_CrCtl_stAccSave,testSig_CrCtl_stCrCUIvLimAdj,testSig_CrCtl_stDecSave,testSig_CrCtl_stStTrans,testSig_CrCtl_stSusp,testSig_CrCtl_rTraV2NBeg_raw,testSig_CrCtl_st_raw,testSig_CrCtl_stSub_raw
  BS_Result : BusSelector  OutputSignals=CrCtl_stAccSave,CrCtl_stCrCUIvLimAdj,CrCtl_stDecSave,CrCtl_stStTrans,CrCtl_stSusp,CrCtl_rTraV2NBeg_raw,CrCtl_st_raw,CrCtl_stSub_raw
  ToWs_Req_Bus_Sig1 : ToWorkspace  VariableName=sig_req_004_001  SaveFormat=Structure With Time
  ToWs_Req_Bus_Sig10 : ToWorkspace  VariableName=sig_req_004_010  SaveFormat=Structure With Time
  ToWs_Req_Bus_Sig11 : ToWorkspace  VariableName=sig_req_004_011  SaveFormat=Structure With Time
  ToWs_Req_Bus_Sig12 : ToWorkspace  VariableName=sig_req_004_012  SaveFormat=Structure With Time
  ToWs_Req_Bus_Sig13 : ToWorkspace  VariableName=sig_req_004_013  SaveFormat=Structure With Time
  ToWs_Req_Bus_Sig14 : ToWorkspace  VariableName=sig_req_004_014  SaveFormat=Structure With Time
  ToWs_Req_Bus_Sig15 : ToWorkspace  VariableName=sig_exp_004_001  SaveFormat=Structure With Time
  ToWs_Req_Bus_Sig16 : ToWorkspace  VariableName=sig_exp_004_002  SaveFormat=Structure With Time
  ToWs_Req_Bus_Sig17 : ToWorkspace  VariableName=sig_exp_004_003  SaveFormat=Structure With Time
  ToWs_Req_Bus_Sig18 : ToWorkspace  VariableName=sig_exp_004_004  SaveFormat=Structure With Time
  ToWs_Req_Bus_Sig19 : ToWorkspace  VariableName=sig_exp_004_005  SaveFormat=Structure With Time
  ToWs_Req_Bus_Sig2 : ToWorkspace  VariableName=sig_req_004_002  SaveFormat=Structure With Time
  ToWs_Req_Bus_Sig20 : ToWorkspace  VariableName=sig_exp_004_006  SaveFormat=Structure With Time
  ToWs_Req_Bus_Sig21 : ToWorkspace  VariableName=sig_exp_004_007  SaveFormat=Structure With Time
  ToWs_Req_Bus_Sig22 : ToWorkspace  VariableName=sig_exp_004_008  SaveFormat=Structure With Time
  ToWs_Req_Bus_Sig3 : ToWorkspace  VariableName=sig_req_004_003  SaveFormat=Structure With Time
  ToWs_Req_Bus_Sig4 : ToWorkspace  VariableName=sig_req_004_004  SaveFormat=Structure With Time
  ToWs_Req_Bus_Sig5 : ToWorkspace  VariableName=sig_req_004_005  SaveFormat=Structure With Time
  ToWs_Req_Bus_Sig6 : ToWorkspace  VariableName=sig_req_004_006  SaveFormat=Structure With Time
  ToWs_Req_Bus_Sig7 : ToWorkspace  VariableName=sig_req_004_007  SaveFormat=Structure With Time
  ToWs_Req_Bus_Sig8 : ToWorkspace  VariableName=sig_req_004_008  SaveFormat=Structure With Time
  ToWs_Req_Bus_Sig9 : ToWorkspace  VariableName=sig_req_004_009  SaveFormat=Structure With Time
  ToWs_Result_Bus_Sig1 : ToWorkspace  VariableName=sig_result_004_001  SaveFormat=Structure With Time
  ToWs_Result_Bus_Sig2 : ToWorkspace  VariableName=sig_result_004_002  SaveFormat=Structure With Time
  ToWs_Result_Bus_Sig3 : ToWorkspace  VariableName=sig_result_004_003  SaveFormat=Structure With Time
  ToWs_Result_Bus_Sig4 : ToWorkspace  VariableName=sig_result_004_004  SaveFormat=Structure With Time
  ToWs_Result_Bus_Sig5 : ToWorkspace  VariableName=sig_result_004_005  SaveFormat=Structure With Time
  ToWs_Result_Bus_Sig6 : ToWorkspace  VariableName=sig_result_004_006  SaveFormat=Structure With Time
  ToWs_Result_Bus_Sig7 : ToWorkspace  VariableName=sig_result_004_007  SaveFormat=Structure With Time
  ToWs_Result_Bus_Sig8 : ToWorkspace  VariableName=sig_result_004_008  SaveFormat=Structure With Time
  specifyOutputs : Subsystem
  result : Outport
  wires:
  sig_Req_Bus/1 -> BS/1, specifyOutputs/1(sig_Req_Bus)
  BS/1 -> ToWs_Req_Bus_Sig1/1  "<testSig_CrCtl_stLck>"
  BS/2 -> ToWs_Req_Bus_Sig2/1  "<testSig_CrCtl_stOpFunc>"
  BS/3 -> ToWs_Req_Bus_Sig3/1  "<testSig_CrCtl_stReq>"
  BS/4 -> ToWs_Req_Bus_Sig4/1  "<testSig_CrCtl_stShOff>"
  BS/5 -> ToWs_Req_Bus_Sig5/1  "<testSig_CrCtl_stSuspAct>"
  BS/6 -> ToWs_Req_Bus_Sig6/1  "<testSig_CrCtl_vDes>"
  BS/7 -> ToWs_Req_Bus_Sig7/1  "<testSig_CrCUI_stBttn>"
  BS/8 -> ToWs_Req_Bus_Sig8/1  "<testSig_GlbDa_vXFlt>"
  BS/9 -> ToWs_Req_Bus_Sig9/1  "<testSig_LLim_stModify>"
  BS/10 -> ToWs_Req_Bus_Sig10/1  "<testSig_PT_rTraV2N>"
  BS/11 -> ToWs_Req_Bus_Sig11/1  "<testSig_WESDem_stCurr>"
  BS/12 -> ToWs_Req_Bus_Sig12/1  "<testSig_CrCtl_st>"
  BS/13 -> ToWs_Req_Bus_Sig13/1  "<testSig_CrCtl_stSub>"
  BS/14 -> ToWs_Req_Bus_Sig14/1  "<testSig_CrCtl_rTraV2NBeg>"
  BS/15 -> ToWs_Req_Bus_Sig15/1  "<testSig_CrCtl_stAccSave>"
  BS/16 -> ToWs_Req_Bus_Sig16/1  "<testSig_CrCtl_stCrCUIvLimAdj>"
  BS/17 -> ToWs_Req_Bus_Sig17/1  "<testSig_CrCtl_stDecSave>"
  BS/18 -> ToWs_Req_Bus_Sig18/1  "<testSig_CrCtl_stStTrans>"
  BS/19 -> ToWs_Req_Bus_Sig19/1  "<testSig_CrCtl_stSusp>"
  BS/20 -> ToWs_Req_Bus_Sig20/1  "<testSig_CrCtl_rTraV2NBeg_raw>"
  BS/21 -> ToWs_Req_Bus_Sig21/1  "<testSig_CrCtl_st_raw>"
  BS/22 -> ToWs_Req_Bus_Sig22/1  "<testSig_CrCtl_stSub_raw>"
  sig_Result_Bus/1 -> BS_Result/1, specifyOutputs/2(sig_Result_Bus)
  BS_Result/1 -> ToWs_Result_Bus_Sig1/1  "<CrCtl_stAccSave>"
  BS_Result/2 -> ToWs_Result_Bus_Sig2/1  "<CrCtl_stCrCUIvLimAdj>"
  BS_Result/3 -> ToWs_Result_Bus_Sig3/1  "<CrCtl_stDecSave>"
  BS_Result/4 -> ToWs_Result_Bus_Sig4/1  "<CrCtl_stStTrans>"
  BS_Result/5 -> ToWs_Result_Bus_Sig5/1  "<CrCtl_stSusp>"
  BS_Result/6 -> ToWs_Result_Bus_Sig6/1  "<CrCtl_rTraV2NBeg_raw>"
  BS_Result/7 -> ToWs_Result_Bus_Sig7/1  "<CrCtl_st_raw>"
  BS_Result/8 -> ToWs_Result_Bus_Sig8/1  "<CrCtl_stSub_raw>"
  specifyOutputs/1(result) -> result/1

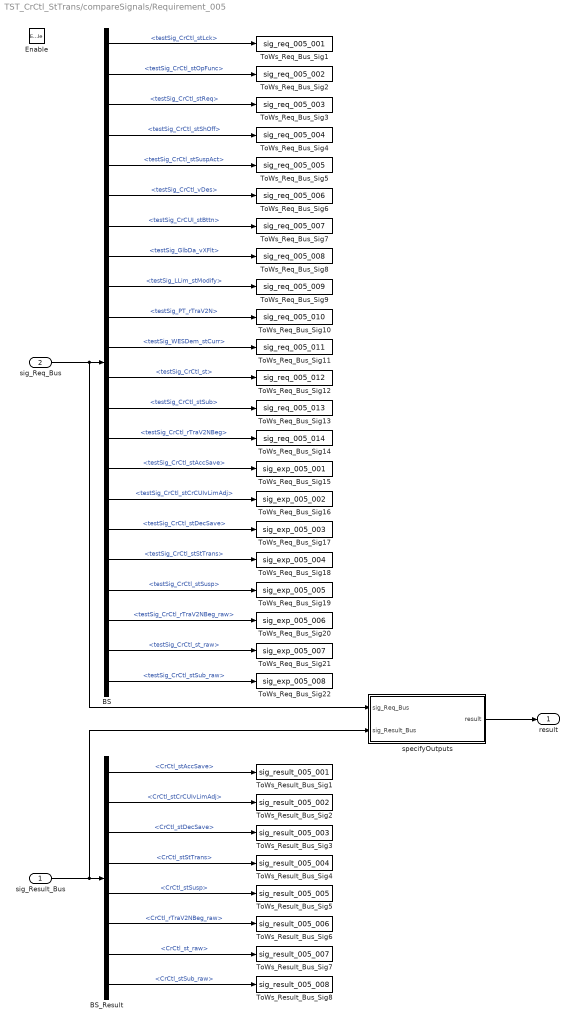
== system TST_CrCtl_StTrans/compareSignals/Requirement_005 ==
  sig_Result_Bus : Inport
  sig_Req_Bus : Inport  Port=2
  Enable : EnablePort
  BS : BusSelector  OutputSignals=testSig_CrCtl_stLck,testSig_CrCtl_stOpFunc,testSig_CrCtl_stReq,testSig_CrCtl_stShOff,testSig_CrCtl_stSuspAct,testSig_CrCtl_vDes,testSig_CrCUI_stBttn,testSig_GlbDa_vXFlt,testSig_LLim_stModify,testSig_PT_rTraV2N,testSig_WESDem_stCurr,testSig_CrCtl_st,testSig_CrCtl_stSub,testSig_CrCtl_rTraV2NBeg,testSig_CrCtl_stAccSave,testSig_CrCtl_stCrCUIvLimAdj,testSig_CrCtl_stDecSave,testSig_CrCtl_stStTrans,testSig_CrCtl_stSusp,testSig_CrCtl_rTraV2NBeg_raw,testSig_CrCtl_st_raw,testSig_CrCtl_stSub_raw
  BS_Result : BusSelector  OutputSignals=CrCtl_stAccSave,CrCtl_stCrCUIvLimAdj,CrCtl_stDecSave,CrCtl_stStTrans,CrCtl_stSusp,CrCtl_rTraV2NBeg_raw,CrCtl_st_raw,CrCtl_stSub_raw
  ToWs_Req_Bus_Sig1 : ToWorkspace  VariableName=sig_req_005_001  SaveFormat=Structure With Time
  ToWs_Req_Bus_Sig10 : ToWorkspace  VariableName=sig_req_005_010  SaveFormat=Structure With Time
  ToWs_Req_Bus_Sig11 : ToWorkspace  VariableName=sig_req_005_011  SaveFormat=Structure With Time
  ToWs_Req_Bus_Sig12 : ToWorkspace  VariableName=sig_req_005_012  SaveFormat=Structure With Time
  ToWs_Req_Bus_Sig13 : ToWorkspace  VariableName=sig_req_005_013  SaveFormat=Structure With Time
  ToWs_Req_Bus_Sig14 : ToWorkspace  VariableName=sig_req_005_014  SaveFormat=Structure With Time
  ToWs_Req_Bus_Sig15 : ToWorkspace  VariableName=sig_exp_005_001  SaveFormat=Structure With Time
  ToWs_Req_Bus_Sig16 : ToWorkspace  VariableName=sig_exp_005_002  SaveFormat=Structure With Time
  ToWs_Req_Bus_Sig17 : ToWorkspace  VariableName=sig_exp_005_003  SaveFormat=Structure With Time
  ToWs_Req_Bus_Sig18 : ToWorkspace  VariableName=sig_exp_005_004  SaveFormat=Structure With Time
  ToWs_Req_Bus_Sig19 : ToWorkspace  VariableName=sig_exp_005_005  SaveFormat=Structure With Time
  ToWs_Req_Bus_Sig2 : ToWorkspace  VariableName=sig_req_005_002  SaveFormat=Structure With Time
  ToWs_Req_Bus_Sig20 : ToWorkspace  VariableName=sig_exp_005_006  SaveFormat=Structure With Time
  ToWs_Req_Bus_Sig21 : ToWorkspace  VariableName=sig_exp_005_007  SaveFormat=Structure With Time
  ToWs_Req_Bus_Sig22 : ToWorkspace  VariableName=sig_exp_005_008  SaveFormat=Structure With Time
  ToWs_Req_Bus_Sig3 : ToWorkspace  VariableName=sig_req_005_003  SaveFormat=Structure With Time
  ToWs_Req_Bus_Sig4 : ToWorkspace  VariableName=sig_req_005_004  SaveFormat=Structure With Time
  ToWs_Req_Bus_Sig5 : ToWorkspace  VariableName=sig_req_005_005  SaveFormat=Structure With Time
  ToWs_Req_Bus_Sig6 : ToWorkspace  VariableName=sig_req_005_006  SaveFormat=Structure With Time
  ToWs_Req_Bus_Sig7 : ToWorkspace  VariableName=sig_req_005_007  SaveFormat=Structure With Time
  ToWs_Req_Bus_Sig8 : ToWorkspace  VariableName=sig_req_005_008  SaveFormat=Structure With Time
  ToWs_Req_Bus_Sig9 : ToWorkspace  VariableName=sig_req_005_009  SaveFormat=Structure With Time
  ToWs_Result_Bus_Sig1 : ToWorkspace  VariableName=sig_result_005_001  SaveFormat=Structure With Time
  ToWs_Result_Bus_Sig2 : ToWorkspace  VariableName=sig_result_005_002  SaveFormat=Structure With Time
  ToWs_Result_Bus_Sig3 : ToWorkspace  VariableName=sig_result_005_003  SaveFormat=Structure With Time
  ToWs_Result_Bus_Sig4 : ToWorkspace  VariableName=sig_result_005_004  SaveFormat=Structure With Time
  ToWs_Result_Bus_Sig5 : ToWorkspace  VariableName=sig_result_005_005  SaveFormat=Structure With Time
  ToWs_Result_Bus_Sig6 : ToWorkspace  VariableName=sig_result_005_006  SaveFormat=Structure With Time
  ToWs_Result_Bus_Sig7 : ToWorkspace  VariableName=sig_result_005_007  SaveFormat=Structure With Time
  ToWs_Result_Bus_Sig8 : ToWorkspace  VariableName=sig_result_005_008  SaveFormat=Structure With Time
  specifyOutputs : Subsystem
  result : Outport
  wires:
  sig_Req_Bus/1 -> BS/1, specifyOutputs/1(sig_Req_Bus)
  BS/1 -> ToWs_Req_Bus_Sig1/1  "<testSig_CrCtl_stLck>"
  BS/2 -> ToWs_Req_Bus_Sig2/1  "<testSig_CrCtl_stOpFunc>"
  BS/3 -> ToWs_Req_Bus_Sig3/1  "<testSig_CrCtl_stReq>"
  BS/4 -> ToWs_Req_Bus_Sig4/1  "<testSig_CrCtl_stShOff>"
  BS/5 -> ToWs_Req_Bus_Sig5/1  "<testSig_CrCtl_stSuspAct>"
  BS/6 -> ToWs_Req_Bus_Sig6/1  "<testSig_CrCtl_vDes>"
  BS/7 -> ToWs_Req_Bus_Sig7/1  "<testSig_CrCUI_stBttn>"
  BS/8 -> ToWs_Req_Bus_Sig8/1  "<testSig_GlbDa_vXFlt>"
  BS/9 -> ToWs_Req_Bus_Sig9/1  "<testSig_LLim_stModify>"
  BS/10 -> ToWs_Req_Bus_Sig10/1  "<testSig_PT_rTraV2N>"
  BS/11 -> ToWs_Req_Bus_Sig11/1  "<testSig_WESDem_stCurr>"
  BS/12 -> ToWs_Req_Bus_Sig12/1  "<testSig_CrCtl_st>"
  BS/13 -> ToWs_Req_Bus_Sig13/1  "<testSig_CrCtl_stSub>"
  BS/14 -> ToWs_Req_Bus_Sig14/1  "<testSig_CrCtl_rTraV2NBeg>"
  BS/15 -> ToWs_Req_Bus_Sig15/1  "<testSig_CrCtl_stAccSave>"
  BS/16 -> ToWs_Req_Bus_Sig16/1  "<testSig_CrCtl_stCrCUIvLimAdj>"
  BS/17 -> ToWs_Req_Bus_Sig17/1  "<testSig_CrCtl_stDecSave>"
  BS/18 -> ToWs_Req_Bus_Sig18/1  "<testSig_CrCtl_stStTrans>"
  BS/19 -> ToWs_Req_Bus_Sig19/1  "<testSig_CrCtl_stSusp>"
  BS/20 -> ToWs_Req_Bus_Sig20/1  "<testSig_CrCtl_rTraV2NBeg_raw>"
  BS/21 -> ToWs_Req_Bus_Sig21/1  "<testSig_CrCtl_st_raw>"
  BS/22 -> ToWs_Req_Bus_Sig22/1  "<testSig_CrCtl_stSub_raw>"
  sig_Result_Bus/1 -> BS_Result/1, specifyOutputs/2(sig_Result_Bus)
  BS_Result/1 -> ToWs_Result_Bus_Sig1/1  "<CrCtl_stAccSave>"
  BS_Result/2 -> ToWs_Result_Bus_Sig2/1  "<CrCtl_stCrCUIvLimAdj>"
  BS_Result/3 -> ToWs_Result_Bus_Sig3/1  "<CrCtl_stDecSave>"
  BS_Result/4 -> ToWs_Result_Bus_Sig4/1  "<CrCtl_stStTrans>"
  BS_Result/5 -> ToWs_Result_Bus_Sig5/1  "<CrCtl_stSusp>"
  BS_Result/6 -> ToWs_Result_Bus_Sig6/1  "<CrCtl_rTraV2NBeg_raw>"
  BS_Result/7 -> ToWs_Result_Bus_Sig7/1  "<CrCtl_st_raw>"
  BS_Result/8 -> ToWs_Result_Bus_Sig8/1  "<CrCtl_stSub_raw>"
  specifyOutputs/1(result) -> result/1

== system TST_CrCtl_StTrans/simulationInput/testSignals_R001 ==
  BC : BusCreator  Inputs=22
  spec_CrCUI_stBttn : FromWorkspace  VariableName=testSig_CrCUI_stBttn  Interpolate=off  OutputAfterFinalValue=Holding final value
  spec_CrCtl_rTraV2NBeg : FromWorkspace  VariableName=testSig_CrCtl_rTraV2NBeg  Interpolate=off  OutputAfterFinalValue=Holding final value
  spec_CrCtl_rTraV2NBeg_raw : FromWorkspace  VariableName=testSig_CrCtl_rTraV2NBeg_raw  Interpolate=off  OutputAfterFinalValue=Holding final value
  spec_CrCtl_st : FromWorkspace  VariableName=testSig_CrCtl_st  Interpolate=off  OutputAfterFinalValue=Holding final value
  spec_CrCtl_stAccSave : FromWorkspace  VariableName=testSig_CrCtl_stAccSave  Interpolate=off  OutputAfterFinalValue=Holding final value
  spec_CrCtl_stCrCUIvLimAdj : FromWorkspace  VariableName=testSig_CrCtl_stCrCUIvLimAdj  Interpolate=off  OutputAfterFinalValue=Holding final value
  spec_CrCtl_stDecSave : FromWorkspace  VariableName=testSig_CrCtl_stDecSave  Interpolate=off  OutputAfterFinalValue=Holding final value
  spec_CrCtl_stLck : FromWorkspace  VariableName=testSig_CrCtl_stLck  Interpolate=off  OutputAfterFinalValue=Holding final value
  spec_CrCtl_stOpFunc : FromWorkspace  VariableName=testSig_CrCtl_stOpFunc  Interpolate=off  OutputAfterFinalValue=Holding final value
  spec_CrCtl_stReq : FromWorkspace  VariableName=testSig_CrCtl_stReq  Interpolate=off  OutputAfterFinalValue=Holding final value
  spec_CrCtl_stShOff : FromWorkspace  VariableName=testSig_CrCtl_stShOff  Interpolate=off  OutputAfterFinalValue=Holding final value
  spec_CrCtl_stStTrans : FromWorkspace  VariableName=testSig_CrCtl_stStTrans  Interpolate=off  OutputAfterFinalValue=Holding final value
  spec_CrCtl_stSub : FromWorkspace  VariableName=testSig_CrCtl_stSub  Interpolate=off  OutputAfterFinalValue=Holding final value
  spec_CrCtl_stSub_raw : FromWorkspace  VariableName=testSig_CrCtl_stSub_raw  Interpolate=off  OutputAfterFinalValue=Holding final value
  spec_CrCtl_stSusp : FromWorkspace  VariableName=testSig_CrCtl_stSusp  Interpolate=off  OutputAfterFinalValue=Holding final value
  spec_CrCtl_stSuspAct : FromWorkspace  VariableName=testSig_CrCtl_stSuspAct  Interpolate=off  OutputAfterFinalValue=Holding final value
  spec_CrCtl_st_raw : FromWorkspace  VariableName=testSig_CrCtl_st_raw  Interpolate=off  OutputAfterFinalValue=Holding final value
  spec_CrCtl_vDes : FromWorkspace  VariableName=testSig_CrCtl_vDes  Interpolate=off  OutputAfterFinalValue=Holding final value
  spec_GlbDa_vXFlt : FromWorkspace  VariableName=testSig_GlbDa_vXFlt  Interpolate=off  OutputAfterFinalValue=Holding final value
  spec_LLim_stModify : FromWorkspace  VariableName=testSig_LLim_stModify  Interpolate=off  OutputAfterFinalValue=Holding final value
  spec_PT_rTraV2N : FromWorkspace  VariableName=testSig_PT_rTraV2N  Interpolate=off  OutputAfterFinalValue=Holding final value
  spec_WESDem_stCurr : FromWorkspace  VariableName=testSig_WESDem_stCurr  Interpolate=off  OutputAfterFinalValue=Holding final value
  testSignals : Outport
  wires:
  BC/1 -> testSignals/1
  spec_CrCtl_stLck/1 -> BC/1  "testSig_CrCtl_stLck"
  spec_CrCtl_stOpFunc/1 -> BC/2  "testSig_CrCtl_stOpFunc"
  spec_CrCtl_stReq/1 -> BC/3  "testSig_CrCtl_stReq"
  spec_CrCtl_stShOff/1 -> BC/4  "testSig_CrCtl_stShOff"
  spec_CrCtl_stSuspAct/1 -> BC/5  "testSig_CrCtl_stSuspAct"
  spec_CrCtl_vDes/1 -> BC/6  "testSig_CrCtl_vDes"
  spec_CrCUI_stBttn/1 -> BC/7  "testSig_CrCUI_stBttn"
  spec_GlbDa_vXFlt/1 -> BC/8  "testSig_GlbDa_vXFlt"
  spec_LLim_stModify/1 -> BC/9  "testSig_LLim_stModify"
  spec_PT_rTraV2N/1 -> BC/10  "testSig_PT_rTraV2N"
  spec_WESDem_stCurr/1 -> BC/11  "testSig_WESDem_stCurr"
  spec_CrCtl_st/1 -> BC/12  "testSig_CrCtl_st"
  spec_CrCtl_stSub/1 -> BC/13  "testSig_CrCtl_stSub"
  spec_CrCtl_rTraV2NBeg/1 -> BC/14  "testSig_CrCtl_rTraV2NBeg"
  spec_CrCtl_stAccSave/1 -> BC/15  "testSig_CrCtl_stAccSave"
  spec_CrCtl_stCrCUIvLimAdj/1 -> BC/16  "testSig_CrCtl_stCrCUIvLimAdj"
  spec_CrCtl_stDecSave/1 -> BC/17  "testSig_CrCtl_stDecSave"
  spec_CrCtl_stStTrans/1 -> BC/18  "testSig_CrCtl_stStTrans"
  spec_CrCtl_stSusp/1 -> BC/19  "testSig_CrCtl_stSusp"
  spec_CrCtl_rTraV2NBeg_raw/1 -> BC/20  "testSig_CrCtl_rTraV2NBeg_raw"
  spec_CrCtl_st_raw/1 -> BC/21  "testSig_CrCtl_st_raw"
  spec_CrCtl_stSub_raw/1 -> BC/22  "testSig_CrCtl_stSub_raw"

== system TST_CrCtl_StTrans/simulationInput/testSignals_R002 ==
  BC : BusCreator  Inputs=22
  spec_CrCUI_stBttn : FromWorkspace  VariableName=testSig_CrCUI_stBttn  Interpolate=off  OutputAfterFinalValue=Holding final value
  spec_CrCtl_rTraV2NBeg : FromWorkspace  VariableName=testSig_CrCtl_rTraV2NBeg  Interpolate=off  OutputAfterFinalValue=Holding final value
  spec_CrCtl_rTraV2NBeg_raw : FromWorkspace  VariableName=testSig_CrCtl_rTraV2NBeg_raw  Interpolate=off  OutputAfterFinalValue=Holding final value
  spec_CrCtl_st : FromWorkspace  VariableName=testSig_CrCtl_st  Interpolate=off  OutputAfterFinalValue=Holding final value
  spec_CrCtl_stAccSave : FromWorkspace  VariableName=testSig_CrCtl_stAccSave  Interpolate=off  OutputAfterFinalValue=Holding final value
  spec_CrCtl_stCrCUIvLimAdj : FromWorkspace  VariableName=testSig_CrCtl_stCrCUIvLimAdj  Interpolate=off  OutputAfterFinalValue=Holding final value
  spec_CrCtl_stDecSave : FromWorkspace  VariableName=testSig_CrCtl_stDecSave  Interpolate=off  OutputAfterFinalValue=Holding final value
  spec_CrCtl_stLck : FromWorkspace  VariableName=testSig_CrCtl_stLck  Interpolate=off  OutputAfterFinalValue=Holding final value
  spec_CrCtl_stOpFunc : FromWorkspace  VariableName=testSig_CrCtl_stOpFunc  Interpolate=off  OutputAfterFinalValue=Holding final value
  spec_CrCtl_stReq : FromWorkspace  VariableName=testSig_CrCtl_stReq  Interpolate=off  OutputAfterFinalValue=Holding final value
  spec_CrCtl_stShOff : FromWorkspace  VariableName=testSig_CrCtl_stShOff  Interpolate=off  OutputAfterFinalValue=Holding final value
  spec_CrCtl_stStTrans : FromWorkspace  VariableName=testSig_CrCtl_stStTrans  Interpolate=off  OutputAfterFinalValue=Holding final value
  spec_CrCtl_stSub : FromWorkspace  VariableName=testSig_CrCtl_stSub  Interpolate=off  OutputAfterFinalValue=Holding final value
  spec_CrCtl_stSub_raw : FromWorkspace  VariableName=testSig_CrCtl_stSub_raw  Interpolate=off  OutputAfterFinalValue=Holding final value
  spec_CrCtl_stSusp : FromWorkspace  VariableName=testSig_CrCtl_stSusp  Interpolate=off  OutputAfterFinalValue=Holding final value
  spec_CrCtl_stSuspAct : FromWorkspace  VariableName=testSig_CrCtl_stSuspAct  Interpolate=off  OutputAfterFinalValue=Holding final value
  spec_CrCtl_st_raw : FromWorkspace  VariableName=testSig_CrCtl_st_raw  Interpolate=off  OutputAfterFinalValue=Holding final value
  spec_CrCtl_vDes : FromWorkspace  VariableName=testSig_CrCtl_vDes  Interpolate=off  OutputAfterFinalValue=Holding final value
  spec_GlbDa_vXFlt : FromWorkspace  VariableName=testSig_GlbDa_vXFlt  Interpolate=off  OutputAfterFinalValue=Holding final value
  spec_LLim_stModify : FromWorkspace  VariableName=testSig_LLim_stModify  Interpolate=off  OutputAfterFinalValue=Holding final value
  spec_PT_rTraV2N : FromWorkspace  VariableName=testSig_PT_rTraV2N  Interpolate=off  OutputAfterFinalValue=Holding final value
  spec_WESDem_stCurr : FromWorkspace  VariableName=testSig_WESDem_stCurr  Interpolate=off  OutputAfterFinalValue=Holding final value
  testSignals : Outport
  wires:
  BC/1 -> testSignals/1
  spec_CrCtl_stLck/1 -> BC/1  "testSig_CrCtl_stLck"
  spec_CrCtl_stOpFunc/1 -> BC/2  "testSig_CrCtl_stOpFunc"
  spec_CrCtl_stReq/1 -> BC/3  "testSig_CrCtl_stReq"
  spec_CrCtl_stShOff/1 -> BC/4  "testSig_CrCtl_stShOff"
  spec_CrCtl_stSuspAct/1 -> BC/5  "testSig_CrCtl_stSuspAct"
  spec_CrCtl_vDes/1 -> BC/6  "testSig_CrCtl_vDes"
  spec_CrCUI_stBttn/1 -> BC/7  "testSig_CrCUI_stBttn"
  spec_GlbDa_vXFlt/1 -> BC/8  "testSig_GlbDa_vXFlt"
  spec_LLim_stModify/1 -> BC/9  "testSig_LLim_stModify"
  spec_PT_rTraV2N/1 -> BC/10  "testSig_PT_rTraV2N"
  spec_WESDem_stCurr/1 -> BC/11  "testSig_WESDem_stCurr"
  spec_CrCtl_st/1 -> BC/12  "testSig_CrCtl_st"
  spec_CrCtl_stSub/1 -> BC/13  "testSig_CrCtl_stSub"
  spec_CrCtl_rTraV2NBeg/1 -> BC/14  "testSig_CrCtl_rTraV2NBeg"
  spec_CrCtl_stAccSave/1 -> BC/15  "testSig_CrCtl_stAccSave"
  spec_CrCtl_stCrCUIvLimAdj/1 -> BC/16  "testSig_CrCtl_stCrCUIvLimAdj"
  spec_CrCtl_stDecSave/1 -> BC/17  "testSig_CrCtl_stDecSave"
  spec_CrCtl_stStTrans/1 -> BC/18  "testSig_CrCtl_stStTrans"
  spec_CrCtl_stSusp/1 -> BC/19  "testSig_CrCtl_stSusp"
  spec_CrCtl_rTraV2NBeg_raw/1 -> BC/20  "testSig_CrCtl_rTraV2NBeg_raw"
  spec_CrCtl_st_raw/1 -> BC/21  "testSig_CrCtl_st_raw"
  spec_CrCtl_stSub_raw/1 -> BC/22  "testSig_CrCtl_stSub_raw"
